simulink model "CM690A_HwAg0Meas"  (R2013b)
settings: Solver=FixedStepDiscrete  SolverMode=SingleTasking  StartTime=0.0  StopTime=22  FixedStep=0.002  RelTol=1e-3
undefined symbols (not defined in the file): ELECGLBPRM_DEGPERREV_DEGPERREV_F32, ELECGLBPRM_HWAGCENTROFFS_HWDEG_F32, ELECGLBPRM_HWAGSATNLOWRLIM_HWDEG_F32, ELECGLBPRM_HWAGSATNUPPRLIM_HWDEG_F32, ELECGLBPRM_HWAGSCA_ULS_F32, ELECGLBPRM_HWAGSPURGEARRAT_ULS_F32, ELECGLBPRM_HWAGSPURTORINGGEARRATSNSR0_ULS_F32, ELECGLBPRM_HWAGSPURTORINGGEARRATSNSR1_ULS_F32, ELECGLBPRM_NOFLT_CNT_U08, ELECGLBPRM_OFFSTRIMNOTPRFMD_CNT_U08, ELECGLBPRM_PRTCLFLT_CNT_U08, ELECGLBPRM_SKIPSTEPFLT_CNT_U08, ELECGLBPRM_SNSRINTFLT_CNT_U08, ELECGLBPRM_VRNRERRFLT_CNT_U08, FLTINJ_HWAG0MEAS_HWAG0, FLTINJ_HWAG0MEAS_TESTOK, HwAg0IfFlt, HwAg0MeasHwAg0IfFltFailStep, HwAg0MeasHwAg0IfFltPassStep, HwAg0MeasHwAg0Snsr0PrtclFltFailStep, HwAg0MeasHwAg0Snsr0PrtclFltPassStep, HwAg0MeasHwAg0Snsr1PrtclFltFailStep, HwAg0MeasHwAg0Snsr1PrtclFltPassStep, HwAg0MeasSnsr0Rev, HwAg0MeasSnsr1Rev, HwAg0MeasStep, HwAg0MeasVrnrErrThd, HwAg0MfgFlt, HwAg0Snsr0PrtclFlt, HwAg0Snsr1PrtclFlt, HWAG10THTOOTHTRIG_CNT_U08, HWAG11THTOOTHTRIG_CNT_U08, NtcSts1, sigbuilder_block, SigQlfr1
libraries: simulink x30, NxtrNvM x3
(part 2 of 5)

== system CM690A_HwAg0Meas/HwAg0Meas/HwAg0MeasPer2 ==
  note: Follow below steps in same order:
      |
      | 1. Check the Sensor Seq Number
      |    1a. Check Sensor Seq Number Logic first
      |    1b. Execute RawHwAgRead
      |    1c. Clear RSENT4CSC = 2046U;
      |    1d. FRS Flag Check: If the RegInpRSENT4FRS==1,  Read the RegInpRSENT4FND
      |
      | Design Note: Registers Read must be done once only. (Pl. see Design Rational Section for detail)
  RegInpRSENT4CS : Inport
  RegInpRSENT4FRXD : Inport  Port=2
  RegInpRSENT4FRS : Inport  Port=3
  RegInpRSENT4FND : Inport  Port=4
  function : TriggerPort  TriggerType=function-call
  Constant : Constant  Value=HWAG10THTOOTHTRIG_CNT_U08
      settings: AttributesFormatString=%<Value>.EngVal = 1
  CopyRight2 : Subsystem  Description=|  mask(Copyright Information){none=on}
      | Copyright info block.                                               
      |                                                                     
      | Place copyright information at the top of every subsystem in design.
      mask prompts: none "No parameters"
      mask help: Place copyright information at the top of every subsystem in design.
      mask Display:
      | NxtrConf = 'Nexteer Confidential';
      | 
      | sys = bdroot; %handle for the current model ("system")
      | first = get_param(sys,'Created');
      | first = first(end-3:end);  %year is last four digits
      | 
      | last = get_param(sys,'LastModifiedDate');
      | if isempty(last)
      |     last = datestr(now,'yyyy');
      | else
      |     last = last(end-3:end);
      | end
      | 
      | if strcmp(first,last)
      |     fprintf('%s -- Copyright %s Nexteer',NxtrConf,first)
      | else
      |     fprintf('%s -- %s%s- %s Nexteer',NxtrConf,char(169),first,last)
      | end
  Data Store Read1 : DataStoreRead  DataStoreName=HwAg0SnsrTrigNr
  If2 : If  RequirementInfo={} %GIDa_6155bf13_cddb_4606_817f_19ff0f92aa5f  NumInputs=2  IfExpression=u1 == u2
  Merge : Merge
  Merge1 : Merge
  Snsr0Read : Subsystem  RequirementInfo={} %GIDa_2ab6b8fe_3fe5_46cd_839a_e0a0bedc927a  TreatAsAtomicUnit=on
  Snsr0Read1 : Subsystem  RequirementInfo={} %GIDa_de6d45b7_1330_48a8_8a4c_631b6b0e9694  TreatAsAtomicUnit=on
  HwAg0Snsr0Raw : Outport
  HwAg0Snsr0TestOk : Outport  Port=2
  wires:
  If2/1 -> Snsr0Read/Action
  RegInpRSENT4CS/1 -> Snsr0Read/1(RegInpRSENT4CS)
  RegInpRSENT4FRXD/1 -> Snsr0Read/2(RegInpRSENT4FRXD)
  RegInpRSENT4FRS/1 -> Snsr0Read/3(RegInpRSENT4FRS)
  RegInpRSENT4FND/1 -> Snsr0Read/4(RegInpRSENT4FND)
  Merge/1 -> HwAg0Snsr0Raw/1
  Merge1/1 -> HwAg0Snsr0TestOk/1
  If2/2 -> Snsr0Read1/Action
  Snsr0Read/1(HwAg0Snsr0Raw) -> Merge/1
  Snsr0Read1/1(HwAg0Snsr0Raw) -> Merge/2
  Snsr0Read/2(HwAg0Snsr0TestOk) -> Merge1/1
  Snsr0Read1/2(HwAg0Snsr0TestOk) -> Merge1/2
  Data Store Read1/1 -> If2/1
  Constant/1 -> If2/2

== system CM690A_HwAg0Meas/HwAg0Meas/HwAg0MeasPer3 ==
  note: Follow below steps in same order:
      |
      | 1. Check the Sensor Seq Number
      |    1a. Check Sensor Seq Number Logic first
      |    1b. Execute RawHwAgRead
      |    1c. Clear RSENT4CSC = 2046U;
      |    1d. FRS Flag Check: If the RegInpRSENT4FRS==1,  Read the RegInpRSENT4FND
      |    1e. SYNCHRONIZATION PULSE Logic
      |
      | Design Note: Registers Read must be done once only. (Pl. see Design Rational Section for detail)
  RegInpRSENT4CS : Inport
  RegInpRSENT4FRXD : Inport  Port=2
  RegInpRSENT4NRS : Inport  Port=3
  RegInpRSENT4FRS : Inport  Port=4
  RegInpRSENT4FND : Inport  Port=5
  function : TriggerPort  TriggerType=function-call
  Constant : Constant  Value=HWAG11THTOOTHTRIG_CNT_U08
      settings: AttributesFormatString=%<Value>.EngVal = 2
  CopyRight2 : Subsystem  Description=|  mask(Copyright Information){none=on}
      | Copyright info block.                                               
      |                                                                     
      | Place copyright information at the top of every subsystem in design.
      mask prompts: none "No parameters"
      mask help: Place copyright information at the top of every subsystem in design.
      mask Display:
      | NxtrConf = 'Nexteer Confidential';
      | 
      | sys = bdroot; %handle for the current model ("system")
      | first = get_param(sys,'Created');
      | first = first(end-3:end);  %year is last four digits
      | 
      | last = get_param(sys,'LastModifiedDate');
      | if isempty(last)
      |     last = datestr(now,'yyyy');
      | else
      |     last = last(end-3:end);
      | end
      | 
      | if strcmp(first,last)
      |     fprintf('%s -- Copyright %s Nexteer',NxtrConf,first)
      | else
      |     fprintf('%s -- %s%s- %s Nexteer',NxtrConf,char(169),first,last)
      | end
  Data Store Read1 : DataStoreRead  DataStoreName=HwAg0SnsrTrigNr
  If1 : If  RequirementInfo={} %GIDa_c79673b4_d970_4e41_9a6f_d8dafcbbb0e1  NumInputs=2  IfExpression=u1 == u2
  Merge : Merge
  Merge1 : Merge
  Snsr1Read : Subsystem  RequirementInfo={} %GIDa_92d913f1_b7bc_4c95_8b6b_3f9b1805b54a  TreatAsAtomicUnit=on
  Snsr1Read1 : Subsystem  RequirementInfo={} %GIDa_e52a39b1_4a11_411e_af63_e5cd3b1f5705  TreatAsAtomicUnit=on
  HwAg0Snsr1Raw1 : Outport
  HwAg0Snsr1TestOk1 : Outport  Port=2
  wires:
  If1/2 -> Snsr1Read1/Action
  If1/1 -> Snsr1Read/Action
  RegInpRSENT4CS/1 -> Snsr1Read/1(RegInpRSENT4CS)
  RegInpRSENT4FRXD/1 -> Snsr1Read/2(RegInpRSENT4FRXD)
  RegInpRSENT4NRS/1 -> Snsr1Read/3(RegInpRSENT4NRS)
  RegInpRSENT4FRS/1 -> Snsr1Read/4(RegInpRSENT4FRS)
  RegInpRSENT4FND/1 -> Snsr1Read/5(RegInpRSENT4FND)
  Snsr1Read/1(HwAg0Snsr1Raw1) -> Merge/1
  Snsr1Read1/1(HwAg0Snsr1Raw) -> Merge/2
  Snsr1Read/2(HwAg0Snsr1TestOk1) -> Merge1/1
  Snsr1Read1/2(HwAg0Snsr1TestOk) -> Merge1/2
  Merge1/1 -> HwAg0Snsr1TestOk1/1
  Merge/1 -> HwAg0Snsr1Raw1/1
  Data Store Read1/1 -> If1/1
  Constant/1 -> If1/2

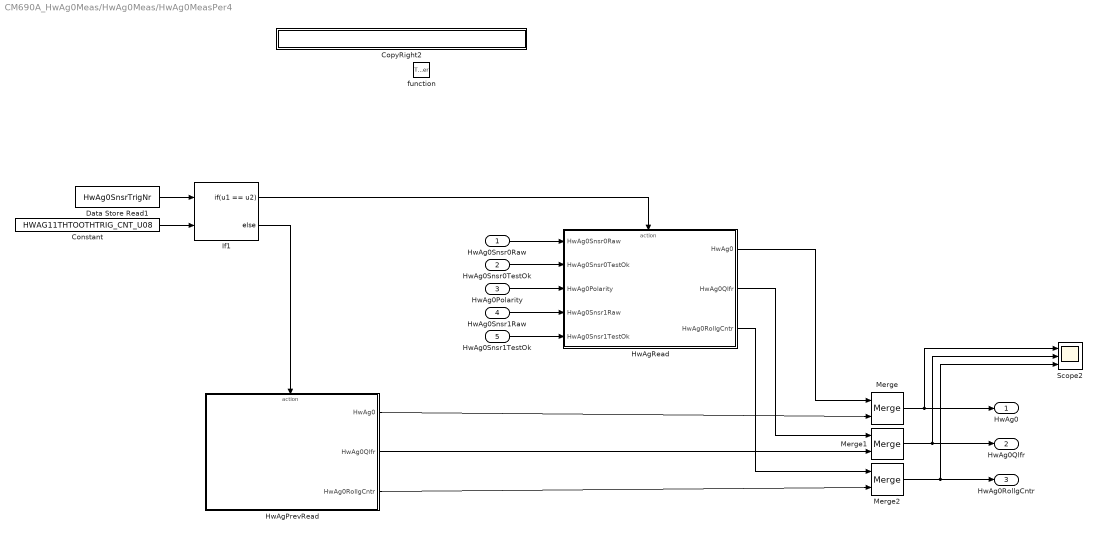
== system CM690A_HwAg0Meas/HwAg0Meas/HwAg0MeasPer4 ==
  HwAg0Snsr0Raw : Inport
  HwAg0Snsr0TestOk : Inport  Port=2
  HwAg0Polarity : Inport  Port=3
  HwAg0Snsr1Raw : Inport  Port=4
  HwAg0Snsr1TestOk : Inport  Port=5
  function : TriggerPort  TriggerType=function-call
  Constant : Constant  Value=HWAG11THTOOTHTRIG_CNT_U08
      settings: AttributesFormatString=%<Value>.EngVal = 2
  CopyRight2 : Subsystem  Description=|  mask(Copyright Information){none=on}
      | Copyright info block.                                               
      |                                                                     
      | Place copyright information at the top of every subsystem in design.
      mask prompts: none "No parameters"
      mask help: Place copyright information at the top of every subsystem in design.
      mask Display:
      | NxtrConf = 'Nexteer Confidential';
      | 
      | sys = bdroot; %handle for the current model ("system")
      | first = get_param(sys,'Created');
      | first = first(end-3:end);  %year is last four digits
      | 
      | last = get_param(sys,'LastModifiedDate');
      | if isempty(last)
      |     last = datestr(now,'yyyy');
      | else
      |     last = last(end-3:end);
      | end
      | 
      | if strcmp(first,last)
      |     fprintf('%s -- Copyright %s Nexteer',NxtrConf,first)
      | else
      |     fprintf('%s -- %s%s- %s Nexteer',NxtrConf,char(169),first,last)
      | end
  Data Store Read1 : DataStoreRead  DataStoreName=HwAg0SnsrTrigNr
  HwAgPrevRead : Subsystem  RequirementInfo={} %GIDa_7375e5dd_6ef3_4731_8150_c23cbc79327b  TreatAsAtomicUnit=on
  HwAgRead : Subsystem  RequirementInfo={} %GIDa_49b889d0_5e4f_426b_aa27_45e0ea96525b  TreatAsAtomicUnit=on
  If1 : If  RequirementInfo={} %GIDa_424aef36_26a1_41c7_8cb5_430e6f82d644  NumInputs=2  IfExpression=u1 == u2
  Merge : Merge
  Merge1 : Merge
  Merge2 : Merge
  Scope2 : Scope  NumInputPorts=3
      settings: TimeRange=22  YMin=-900~0~1  YMax=900~275~2  SaveName=ScopeData6
  HwAg0 : Outport  RequirementInfo={} %GIDa_a55d0ad3_e601_49c7_b914_9c4e7bab7fda
  HwAg0Qlfr : Outport  RequirementInfo={'linktype_rmi_doors' '0000cf45 (/ESG Group/FDD Module Requirements/EA4 Specific/CM690A_HwAg0Meas)' '#CM690A_30' 'true' 'REQ: CM690A_30' '' } %GIDa_08dc6d09_800d_4647_82e3_4af412467949  Port=2
  HwAg0RollgCntr : Outport  RequirementInfo={'linktype_rmi_doors' '0000cf45 (/ESG Group/FDD Module Requirements/EA4 Specific/CM690A_HwAg0Meas)' '#CM690A_31' 'true' 'REQ: CM690A_31' '' } %GIDa_3c51bdf7_5d2b_4414_9b3f_5b588ccc6872  Port=3
  wires:
  If1/2 -> HwAgPrevRead/Action
  If1/1 -> HwAgRead/Action
  HwAgRead/1(HwAg0) -> Merge/1
  HwAgPrevRead/1(HwAg0) -> Merge/2
  HwAgRead/2(HwAg0Qlfr) -> Merge1/1
  HwAgPrevRead/2(HwAg0Qlfr) -> Merge1/2
  HwAgPrevRead/3(HwAg0RollgCntr) -> Merge2/2
  HwAgRead/3(HwAg0RollgCntr) -> Merge2/1
  Merge/1 -> Scope2/1, HwAg0/1
  Merge1/1 -> Scope2/2, HwAg0Qlfr/1
  Merge2/1 -> Scope2/3, HwAg0RollgCntr/1
  HwAg0Snsr1Raw/1 -> HwAgRead/4(HwAg0Snsr1Raw)
  HwAg0Polarity/1 -> HwAgRead/3(HwAg0Polarity)
  HwAg0Snsr1TestOk/1 -> HwAgRead/5(HwAg0Snsr1TestOk)
  HwAg0Snsr0TestOk/1 -> HwAgRead/2(HwAg0Snsr0TestOk)
  HwAg0Snsr0Raw/1 -> HwAgRead/1(HwAg0Snsr0Raw)
  Data Store Read1/1 -> If1/1
  Constant/1 -> If1/2

== system CM690A_HwAg0Meas/HwAg0Meas/HwAg0MeasPer5 ==
  note: Information Only:
      | - Trim not performed Ntc
  function : TriggerPort  TriggerType=function-call
  Constant : Constant  Value=HwAg0MfgFlt
  CopyRight2 : Subsystem  Description=|  mask(Copyright Information){none=on}
      | Copyright info block.                                               
      |                                                                     
      | Place copyright information at the top of every subsystem in design.
      mask prompts: none "No parameters"
      mask help: Place copyright information at the top of every subsystem in design.
      mask Display:
      | NxtrConf = 'Nexteer Confidential';
      | 
      | sys = bdroot; %handle for the current model ("system")
      | first = get_param(sys,'Created');
      | first = first(end-3:end);  %year is last four digits
      | 
      | last = get_param(sys,'LastModifiedDate');
      | if isempty(last)
      |     last = datestr(now,'yyyy');
      | else
      |     last = last(end-3:end);
      | end
      | 
      | if strcmp(first,last)
      |     fprintf('%s -- Copyright %s Nexteer',NxtrConf,first)
      | else
      |     fprintf('%s -- %s%s- %s Nexteer',NxtrConf,char(169),first,last)
      | end
  Data Store Read1 : DataStoreRead  DataStoreName=HwAg0OffsTrimPrfmdSts
  Ground : Ground
  If : If  IfExpression=(u1 ~= 0)
  If Action Subsystem : Subsystem  RequirementInfo={'linktype_rmi_doors' '0000cf45 (/ESG Group/FDD Module Requirements/EA4 Specific/CM690A_HwAg0Meas)' '#CM690A_107' 'true' 'REQ: CM690A_107' '' } %GIDa_93c0c2f6_38ee_4160_b051_f0ab663f9dc9  TreatAsAtomicUnit=on
  If Action Subsystem1 : Subsystem  RequirementInfo={'linktype_rmi_doors' '0000cf45 (/ESG Group/FDD Module Requirements/EA4 Specific/CM690A_HwAg0Meas)' '#CM690A_104' 'true' 'REQ: CM690A_104' '' } %GIDa_fa6d762f_0a06_4ac8_8aec_4f8d74e26f90  TreatAsAtomicUnit=on
  Merge : Merge
  Merge1 : Merge
  Scope : Scope  NumInputPorts=2
      settings: YMin=-5~-5  YMax=5~5  SaveName=ScopeData3
  SetNtcSts : Subsystem  RequirementInfo={'linktype_rmi_doors' '0000cf45 (/ESG Group/FDD Module Requirements/EA4 Specific/CM690A_HwAg0Meas)' '#CM690A_100' 'true' 'REQ: CM690A_100' '' } %GIDa_9e3edb63_7888_44cf_a718_771f9129b5ad
  wires:
  Ground/1 -> SetNtcSts/4(DebStep)
  Constant/1 -> SetNtcSts/1(NtcNr)
  Data Store Read1/1 -> If/1
  If/1 -> If Action Subsystem/Action
  If/2 -> If Action Subsystem1/Action
  If Action Subsystem/1(ParamByte) -> Merge/1
  If Action Subsystem1/1(ParamByte) -> Merge/2
  If Action Subsystem/2(TestOk) -> Merge1/1
  If Action Subsystem1/2(TestOk) -> Merge1/2
  Merge/1 -> Scope/1, SetNtcSts/2(NtcStInfo)  "ParamByte"
  Merge1/1 -> Scope/2, SetNtcSts/3(NtcSts)  "TestOk"

== system CM690A_HwAg0Meas/Simulated_Input/CopyRight2 ==

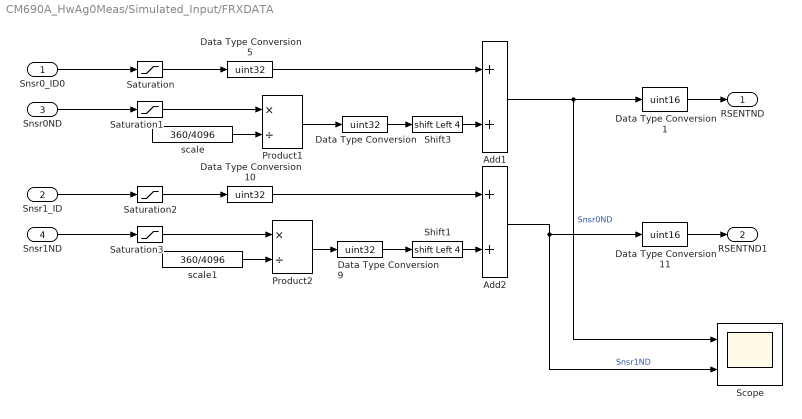
== system CM690A_HwAg0Meas/Simulated_Input/FRXDATA ==
  Snsr0_ID0 : Inport
  Snsr1_ID : Inport  Port=2
  Snsr0ND : Inport  Port=3
  Snsr1ND : Inport  Port=4
  Add1 : Sum
  Add2 : Sum
  Data Type Conversion : DataTypeConversion  OutDataTypeStr=uint32
  Data Type Conversion1 : DataTypeConversion  OutDataTypeStr=uint16
  Data Type Conversion10 : DataTypeConversion  OutDataTypeStr=uint32  SaturateOnIntegerOverflow=on
  Data Type Conversion11 : DataTypeConversion  OutDataTypeStr=uint16
  Data Type Conversion5 : DataTypeConversion  OutDataTypeStr=uint32
  Data Type Conversion9 : DataTypeConversion  OutDataTypeStr=uint32
  Product1 : Product  Inputs=*/
  Product2 : Product  Inputs=*/
  Saturation : Saturate  UpperLimit=1  LowerLimit=0
  Saturation1 : Saturate  UpperLimit=360  LowerLimit=0
  Saturation2 : Saturate  UpperLimit=1  LowerLimit=0
  Saturation3 : Saturate  UpperLimit=360  LowerLimit=0
  Scope : Scope  NumInputPorts=2
      settings: YMin=1.02005e+09~0  YMax=1.12743e+09~6e+08
  Shift1 : ArithShift  BitShiftNumber=4  BitShiftDirection=Left
  Shift3 : ArithShift  BitShiftNumber=4  BitShiftDirection=Left
  scale : Constant  Value=360/4096
  scale1 : Constant  Value=360/4096
  RSENTND : Outport
  RSENTND1 : Outport  Port=2
  wires:
  Snsr0ND/1 -> Saturation1/1
  scale/1 -> Product1/2
  Product1/1 -> Data Type Conversion/1
  Data Type Conversion1/1 -> RSENTND/1
  Snsr0_ID0/1 -> Saturation/1
  Data Type Conversion5/1 -> Add1/1
  Data Type Conversion/1 -> Shift3/1
  Add1/1 -> Scope/1, Data Type Conversion1/1  "Snsr0ND"
  Snsr1ND/1 -> Saturation3/1
  scale1/1 -> Product2/2
  Product2/1 -> Data Type Conversion9/1
  Snsr1_ID/1 -> Saturation2/1
  Data Type Conversion10/1 -> Add2/1
  Data Type Conversion9/1 -> Shift1/1
  Data Type Conversion11/1 -> RSENTND1/1
  Add2/1 -> Data Type Conversion11/1, Scope/2  "Snsr1ND"
  Saturation/1 -> Data Type Conversion5/1
  Saturation1/1 -> Product1/1
  Saturation2/1 -> Data Type Conversion10/1
  Saturation3/1 -> Product2/1
  Shift3/1 -> Add1/2
  Shift1/1 -> Add2/2

== system CM690A_HwAg0Meas/Simulated_Input/FRXDATA1 ==
  Snsr0_CS : Inport
  Snsr1_CS : Inport  Port=2
  Snsr0_FRS : Inport  Port=3
  Snsr1_FRS : Inport  Port=4
  Add1 : Sum
  Add2 : Sum
  Data Type Conversion{,1,5,9,11} (5 alike) : DataTypeConversion  OutDataTypeStr=uint32
  Data Type Conversion10 : DataTypeConversion  OutDataTypeStr=uint32  SaturateOnIntegerOverflow=on
  Scope : Scope  NumInputPorts=2
      settings: YMin=1.02005e+09~0  YMax=1.12743e+09~6e+08
  Shift1 : ArithShift  BitShiftNumber=1  BitShiftDirection=Left
  Shift3 : ArithShift  BitShiftNumber=1  BitShiftDirection=Left
  Snsr0CS : Outport
  Snsr1CS : Outport  Port=2
  wires:
  Data Type Conversion9/1 -> Add2/2
  Data Type Conversion/1 -> Add1/2
  Snsr1_CS/1 -> Data Type Conversion10/1
  Snsr0_CS/1 -> Data Type Conversion5/1
  Add2/1 -> Scope/2, Data Type Conversion11/1  "Snsr1ND"
  Data Type Conversion11/1 -> Snsr1CS/1
  Data Type Conversion10/1 -> Shift1/1
  Add1/1 -> Data Type Conversion1/1, Scope/1  "Snsr0ND"
  Data Type Conversion5/1 -> Shift3/1
  Data Type Conversion1/1 -> Snsr0CS/1
  Snsr0_FRS/1 -> Data Type Conversion/1
  Snsr1_FRS/1 -> Data Type Conversion9/1
  Shift3/1 -> Add1/1
  Shift1/1 -> Add2/1

== system CM690A_HwAg0Meas/Simulated_Input/FRXDATA2 ==
  Snsr0_FCCN : Inport
  Snsr1_FCCN : Inport  Port=2
  Snsr0_Data : Inport  Port=3
  Snsr1_Data : Inport  Port=4
  Add1 : Sum
  Add2 : Sum
  Data Type Conversion{,1,5,9,11} (5 alike) : DataTypeConversion  OutDataTypeStr=uint32
  Data Type Conversion10 : DataTypeConversion  OutDataTypeStr=uint32  SaturateOnIntegerOverflow=on
  Scope : Scope  NumInputPorts=2
      settings: YMin=1.02005e+09~0  YMax=1.12743e+09~6e+08
  Shift1 : ArithShift  BitShiftNumber=28  BitShiftDirection=Left
  Shift3 : ArithShift  BitShiftNumber=28  BitShiftDirection=Left
  Snsr0FRXD : Outport
  Snsr1FRXD : Outport  Port=2
  wires:
  Shift1/1 -> Add2/1
  Shift3/1 -> Add1/1
  Snsr1_Data/1 -> Data Type Conversion9/1
  Snsr0_Data/1 -> Data Type Conversion/1
  Data Type Conversion1/1 -> Snsr0FRXD/1
  Data Type Conversion5/1 -> Shift3/1
  Add1/1 -> Scope/1, Data Type Conversion1/1  "Snsr0ND"
  Data Type Conversion10/1 -> Shift1/1
  Data Type Conversion11/1 -> Snsr1FRXD/1
  Add2/1 -> Data Type Conversion11/1, Scope/2  "Snsr1ND"
  Snsr0_FCCN/1 -> Data Type Conversion5/1
  Snsr1_FCCN/1 -> Data Type Conversion10/1
  Data Type Conversion/1 -> Add1/2
  Data Type Conversion9/1 -> Add2/2

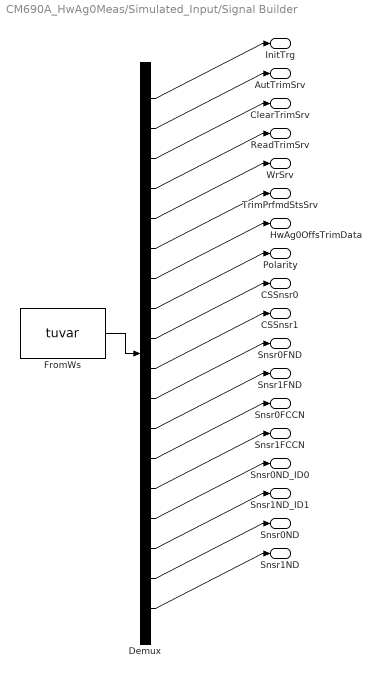
== system CM690A_HwAg0Meas/Simulated_Input/Signal Builder ==
  Demux : Demux  Tag=STV Demux  Outputs=18
  FromWs : FromWorkspace  Tag=STV FromWs  VariableName=tuvar  SampleTime=0  OutputAfterFinalValue=Holding final value
      SigBuilderData=|
      | common.afterFinalStr = 'Hold final value'
      | common.sampleTime = '0'
      | dataSet(1).timeRange = [0 22]
      | dataSet(1).name = 'IdealSignal'
      | dataSet(2).timeRange = [0 22]
      | dataSet(2).name = 'Faults'
      | dataSet(3).timeRange = [0 22]
      | dataSet(3).name = 'Service'
      | dataSet(4).timeRange = [0 22]
      | dataSet(4).name = 'RollOver'
      | sbobj.Groups(1).Name = 'IdealSignal'
      | sbobj.Groups(1).Signals(1).Name = 'InitTrg'
      | sbobj.Groups(1).Signals(1).XData = [0 0.02 0.02 0.06 0.06 22]
      | sbobj.Groups(1).Signals(1).YData = [0 0 1 1 0 0]
      | sbobj.Groups(1).Signals(2).Name = 'AutTrimSrv'
      | sbobj.Groups(1).Signals(2).XData = [0 22]
      | sbobj.Groups(1).Signals(2).YData = [0 0]
      | sbobj.Groups(1).Signals(3).Name = 'ClearTrimSrv'
      | sbobj.Groups(1).Signals(3).XData = [0 22]
      | sbobj.Groups(1).Signals(3).YData = [0 0]
      | sbobj.Groups(1).Signals(4).Name = 'ReadTrimSrv'
      | sbobj.Groups(1).Signals(4).XData = [0 22]
      | sbobj.Groups(1).Signals(4).YData = [0 0]
      | sbobj.Groups(1).Signals(5).Name = 'WrSrv'
      | sbobj.Groups(1).Signals(5).XData = [0 0.04 0.04 0.08 0.08 22]
      | sbobj.Groups(1).Signals(5).YData = [0 0 1 1 0 0]
      | sbobj.Groups(1).Signals(6).Name = 'TrimPrfmdStsSrv'
      | sbobj.Groups(1).Signals(6).XData = [0 22]
      | sbobj.Groups(1).Signals(6).YData = [0 0]
      | sbobj.Groups(1).Signals(7).Name = 'HwAg0OffsTrimData'
      | sbobj.Groups(1).Signals(7).XData = [0 22]
      | sbobj.Groups(1).Signals(7).YData = [0 0]
      | sbobj.Groups(1).Signals(8).Name = 'Polarity'
      | sbobj.Groups(1).Signals(8).XData = [0 22]
      | sbobj.Groups(1).Signals(8).YData = [1 1]
      | sbobj.Groups(1).Signals(9).Name = 'CSSnsr0'
      | sbobj.Groups(1).Signals(9).XData = [0 22]
      | sbobj.Groups(1).Signals(9).YData = [0 0]
      | sbobj.Groups(1).Signals(10).Name = 'CSSnsr1'
      | sbobj.Groups(1).Signals(10).XData = [0 22]
      | sbobj.Groups(1).Signals(10).YData = [0 0]
      | sbobj.Groups(1).Signals(11).Name = 'Snsr0FND'
      | sbobj.Groups(1).Signals(11).XData = [0 22]
      | sbobj.Groups(1).Signals(11).YData = [1 1]
      | sbobj.Groups(1).Signals(12).Name = 'Snsr1FND'
      | sbobj.Groups(1).Signals(12).XData = [0 22]
      | sbobj.Groups(1).Signals(12).YData = [1 1]
      | sbobj.Groups(1).Signals(13).Name = 'Snsr0FCCN'
      | sbobj.Groups(1).Signals(13).XData = [0 22]
      | sbobj.Groups(1).Signals(13).YData = [0 0]
      | sbobj.Groups(1).Signals(14).Name = 'Snsr1FCCN'
      | sbobj.Groups(1).Signals(14).XData = [0 22]
      | sbobj.Groups(1).Signals(14).YData = [0 0]
      | sbobj.Groups(1).Signals(15).Name = 'Snsr0ND_ID0'
      | sbobj.Groups(1).Signals(15).XData = [0 22]
      | sbobj.Groups(1).Signals(15).YData = [0 0]
      | sbobj.Groups(1).Signals(16).Name = 'Snsr1ND_ID1'
      | sbobj.Groups(1).Signals(16).XData = [0 22]
      | sbobj.Groups(1).Signals(16).YData = [1 1]
      | sbobj.Groups(1).Signals(17).Name = 'Snsr0ND'
      | sbobj.Groups(1).Signals(17).XData = [0 2 2 4 4 6 6 8 8 10 10 12 12 14 14 16 16 18 18 20 20 22]
      | sbobj.Groups(1).Signals(17).YData = [0 359.9 0 359.9 0 359.9 0 359.9 0 359.9 0 359.9 0 359.9 0 359.9 0 359.9 0 359.9 0 359.9]
      | sbobj.Groups(1).Signals(18).Name = 'Snsr1ND'
      | sbobj.Groups(1).Signals(18).XData = [0 2.2000022 2.2000022 4.4000044 4.4000044 6.60000660001 6.60000660001 8.80000880001 8.80000880001 11.000011 11.000011 13.2000132 13.2000132 15.4000154 15.4000154 17.6000176 17.6000176 19.8000198 19.8000198 22]
      | sbobj.Groups(1).Signals(18).YData = [0 359.9 0 359.9 0 359.9 0 359.9 0 359.9 0 359.9 0 359.9 0 359.9 0 359.9 0 359.896401]
      | sbobj.Groups(1).TimeRange = [0 22]
      | sbobj.Groups(2).Name = 'Faults'
      | sbobj.Groups(2).Signals(1).Name = 'InitTrg'
      | sbobj.Groups(2).Signals(1).XData = [0 0.02 0.02 0.06 0.06 22]
      | sbobj.Groups(2).Signals(1).YData = [0 0 1 1 0 0]
      | sbobj.Groups(2).Signals(2).Name = 'AutTrimSrv'
      | sbobj.Groups(2).Signals(2).XData = [0 22]
      | sbobj.Groups(2).Signals(2).YData = [0 0]
      | sbobj.Groups(2).Signals(3).Name = 'ClearTrimSrv'
      | sbobj.Groups(2).Signals(3).XData = [0 22]
      | sbobj.Groups(2).Signals(3).YData = [0 0]
      | sbobj.Groups(2).Signals(4).Name = 'ReadTrimSrv'
      | sbobj.Groups(2).Signals(4).XData = [0 22]
      | sbobj.Groups(2).Signals(4).YData = [0 0]
      | sbobj.Groups(2).Signals(5).Name = 'WrSrv'
      | sbobj.Groups(2).Signals(5).XData = [0 0.06 0.06 0.12 0.12 22]
      | sbobj.Groups(2).Signals(5).YData = [0 0 1 1 0 0]
      | sbobj.Groups(2).Signals(6).Name = 'TrimPrfmdStsSrv'
      | sbobj.Groups(2).Signals(6).XData = [0 22]
      | sbobj.Groups(2).Signals(6).YData = [0 0]
      | sbobj.Groups(2).Signals(7).Name = 'HwAg0OffsTrimData'
      | sbobj.Groups(2).Signals(7).XData = [0 22]
      | sbobj.Groups(2).Signals(7).YData = [0 0]
      | sbobj.Groups(2).Signals(8).Name = 'Polarity'
      | sbobj.Groups(2).Signals(8).XData = [0 11 11 22]
      | sbobj.Groups(2).Signals(8).YData = [-1 -1 1 1]
      | sbobj.Groups(2).Signals(9).Name = 'CSSnsr0'
      | sbobj.Groups(2).Signals(9).XData = [0 2.54 2.54 2.88 2.88 22]
      | sbobj.Groups(2).Signals(9).YData = [0 0 2 2 0 0]
      | sbobj.Groups(2).Signals(10).Name = 'CSSnsr1'
      | sbobj.Groups(2).Signals(10).XData = [0 4.36 4.36 4.78 4.78 22]
      | sbobj.Groups(2).Signals(10).YData = [0 0 2 2 0 0]
      | sbobj.Groups(2).Signals(11).Name = 'Snsr0FND'
      | sbobj.Groups(2).Signals(11).XData = [0 14.54 14.54 14.78 14.78 22]
      | sbobj.Groups(2).Signals(11).YData = [1 1 0 0 1 1]
      | sbobj.Groups(2).Signals(12).Name = 'Snsr1FND'
      | sbobj.Groups(2).Signals(12).XData = [0 15.66 15.66 15.94 15.94 22]
      | sbobj.Groups(2).Signals(12).YData = [1 1 0 0 1 1]
      | sbobj.Groups(2).Signals(13).Name = 'Snsr0FCCN'
      | sbobj.Groups(2).Signals(13).XData = [0 12.02 12.02 12.26 12.26 22]
      | sbobj.Groups(2).Signals(13).YData = [0 0 1 1 0 0]
      | sbobj.Groups(2).Signals(14).Name = 'Snsr1FCCN'
      | sbobj.Groups(2).Signals(14).XData = [0 12.92 12.92 13.2 13.2 22]
      | sbobj.Groups(2).Signals(14).YData = [0 0 2 2 0 0]
      | sbobj.Groups(2).Signals(15).Name = 'Snsr0ND_ID0'
      | sbobj.Groups(2).Signals(15).XData = [0 6.46 6.46 6.8 6.8 22]
      | sbobj.Groups(2).Signals(15).YData = [0 0 1 1 0 0]
      | sbobj.Groups(2).Signals(16).Name = 'Snsr1ND_ID1'
      | sbobj.Groups(2).Signals(16).XData = [0 8.8 8.8 9.32 9.32 22]
      | sbobj.Groups(2).Signals(16).YData = [1 1 0 0 1 1]
      | sbobj.Groups(2).Signals(17).Name = 'Snsr0ND'
      | sbobj.Groups(2).Signals(17).XData = [0 2 2 4 4 6 6 8 8 10 10 12 12 14 14 16 16 18 18 20 20 22]
      | sbobj.Groups(2).Signals(17).YData = [0 359.9 0 359.9 0 359.9 0 359.9 0 359.9 0 359.9 0 359.9 0 359.9 0 359.9 0 359.9 0 350]
      | sbobj.Groups(2).Signals(18).Name = 'Snsr1ND'
      | sbobj.Groups(2).Signals(18).XData = [0 2.2000022 2.2000022 4.4000044 4.4000044 6.60000660001 6.60000660001 8.80000880001 8.80000880001 11.000011 11.000011 13.2000132 13.2000132 15.4000154 15.4000154 17.6000176 17.6000176 20 20 22]
      | sbobj.Groups(2).Signals(18).YData = [0 359.9 0 359.9 0 359.9 0 359.9 0 359.9 0 359.9 0 359.9 0 359.9 0 359.9 0 350]
      | sbobj.Groups(2).TimeRange = [0 22]
      | sbobj.Groups(3).Name = 'Service'
      | sbobj.Groups(3).Signals(1).Name = 'InitTrg'
      | sbobj.Groups(3).Signals(1).XData = [0 0.02 0.02 0.06 0.06 22]
      | sbobj.Groups(3).Signals(1).YData = [0 0 1 1 0 0]
      | sbobj.Groups(3).Signals(2).Name = 'AutTrimSrv'
      | sbobj.Groups(3).Signals(2).XData = [0 0.58 0.58 0.68 0.68 16 16 16.1 16.1 22]
      | sbobj.Groups(3).Signals(2).YData = [0 0 1 1 0 0 1 1 0 0]
      | sbobj.Groups(3).Signals(3).Name = 'ClearTrimSrv'
      | sbobj.Groups(3).Signals(3).XData = [0 0.34 4.1 4.1 4.16 4.16 9.98 9.98 10.06 10.06 22]
      | sbobj.Groups(3).Signals(3).YData = [0 0 0 1 1 0 0 1 1 0 0]
      | sbobj.Groups(3).Signals(4).Name = 'ReadTrimSrv'
      | sbobj.Groups(3).Signals(4).XData = [0 1.24 1.24 1.32 1.32 4.62 4.62 4.7 4.7 6.84 6.84 6.92 6.92 10.38 10.38 10.46 10.46 16.72 16.72 16.8 16.8 22]
      | sbobj.Groups(3).Signals(4).YData = [0 0 1 1 0 0 1 1 0 0 1 1 0 0 1 1 0 0 1 1 0 0]
      | sbobj.Groups(3).Signals(5).Name = 'WrSrv'
      | sbobj.Groups(3).Signals(5).XData = [0 6.22 6.22 6.3 6.3 22]
      | sbobj.Groups(3).Signals(5).YData = [0 0 1 1 0 0]
      | sbobj.Groups(3).Signals(6).Name = 'TrimPrfmdStsSrv'
      | sbobj.Groups(3).Signals(6).XData = [0 1.24 1.24 1.32 1.32 4.64 4.64 4.7 4.7 6.84 6.84 6.92 6.92 10.64 10.64 10.72 10.72 16.74 16.74 16.82 16.82 22]
      | sbobj.Groups(3).Signals(6).YData = [0 0 1 1 0 0 1 1 0 0 1 1 0 0 1 1 0 0 1 1 0 0]
      | sbobj.Groups(3).Signals(7).Name = 'HwAg0OffsTrimData'
      | sbobj.Groups(3).Signals(7).XData = [0 0.4 5.4 5.4 11.16 11.16 22]
      | sbobj.Groups(3).Signals(7).YData = [0 0 0 300 300 0 0]
      | sbobj.Groups(3).Signals(8).Name = 'Polarity'
      | sbobj.Groups(3).Signals(8).XData = [0 22]
      | sbobj.Groups(3).Signals(8).YData = [1 1]
      | sbobj.Groups(3).Signals(9).Name = 'CSSnsr0'
      | sbobj.Groups(3).Signals(9).XData = [0 22]
      | sbobj.Groups(3).Signals(9).YData = [0 0]
      | sbobj.Groups(3).Signals(10).Name = 'CSSnsr1'
      | sbobj.Groups(3).Signals(10).XData = [0 22]
      | sbobj.Groups(3).Signals(10).YData = [0 0]
      | sbobj.Groups(3).Signals(11).Name = 'Snsr0FND'
      | sbobj.Groups(3).Signals(11).XData = [0 22]
      | sbobj.Groups(3).Signals(11).YData = [1 1]
      | sbobj.Groups(3).Signals(12).Name = 'Snsr1FND'
      | sbobj.Groups(3).Signals(12).XData = [0 22]
      | sbobj.Groups(3).Signals(12).YData = [1 1]
      | sbobj.Groups(3).Signals(13).Name = 'Snsr0FCCN'
      | sbobj.Groups(3).Signals(13).XData = [0 22]
      | sbobj.Groups(3).Signals(13).YData = [0 0]
      | sbobj.Groups(3).Signals(14).Name = 'Snsr1FCCN'
      | sbobj.Groups(3).Signals(14).XData = [0 22]
      | sbobj.Groups(3).Signals(14).YData = [0 0]
      | sbobj.Groups(3).Signals(15).Name = 'Snsr0ND_ID0'
      | sbobj.Groups(3).Signals(15).XData = [0 22]
      | sbobj.Groups(3).Signals(15).YData = [0 0]
      | sbobj.Groups(3).Signals(16).Name = 'Snsr1ND_ID1'
      | sbobj.Groups(3).Signals(16).XData = [0 22]
      | sbobj.Groups(3).Signals(16).YData = [1 1]
      | sbobj.Groups(3).Signals(17).Name = 'Snsr0ND'
      | sbobj.Groups(3).Signals(17).XData = [0 2 2 4 4 6 6 8 8 10 10 12 12 14 14 16 16 18 18 20 20 22]
      | sbobj.Groups(3).Signals(17).YData = [0 359.9 0 359.9 0 359.9 0 359.9 0 359.9 0 359.9 0 359.9 0 359.9 0 359.9 0 359.9 0 359.9]
      | sbobj.Groups(3).Signals(18).Name = 'Snsr1ND'
      | sbobj.Groups(3).Signals(18).XData = [0 2.2000022 2.2000022 4.4000044 4.4000044 6.60000660001 6.60000660001 8.80000880001 8.80000880001 11.000011 11.000011 13.2000132 13.2000132 15.4000154 15.4000154 17.6000176 17.6000176 19.8000198 19.8000198 22]
      | sbobj.Groups(3).Signals(18).YData = [0 359.9 0 359.9 0 359.9 0 359.9 0 359.9 0 359.9 0 359.9 0 359.9 0 359.9 0 359.896401]
      | sbobj.Groups(3).TimeRange = [0 22]
      | sbobj.Groups(4).Name = 'RollOver'
      | sbobj.Groups(4).Signals(1).Name = 'InitTrg'
      | sbobj.Groups(4).Signals(1).XData = [0 0.02 0.02 0.06 0.06 22]
      | sbobj.Groups(4).Signals(1).YData = [0 0 1 1 0 0]
      | sbobj.Groups(4).Signals(2).Name = 'AutTrimSrv'
      | sbobj.Groups(4).Signals(2).XData = [0 0.58 0.58 0.68 0.68 15.76 16.1 22]
      | sbobj.Groups(4).Signals(2).YData = [0 0 1 1 0 0 0 0]
      | sbobj.Groups(4).Signals(3).Name = 'ClearTrimSrv'
      | sbobj.Groups(4).Signals(3).XData = [0 22]
      | sbobj.Groups(4).Signals(3).YData = [0 0]
      | sbobj.Groups(4).Signals(4).Name = 'ReadTrimSrv'
      | sbobj.Groups(4).Signals(4).XData = [0 1.24 1.24 1.32 1.32 4.62 4.62 4.7 4.7 6.84 6.84 6.92 6.92 10.38 10.38 10.46 10.46 16.72 16.72 16.8 16.8 22]
      | sbobj.Groups(4).Signals(4).YData = [0 0 1 1 0 0 1 1 0 0 1 1 0 0 1 1 0 0 1 1 0 0]
      | sbobj.Groups(4).Signals(5).Name = 'WrSrv'
      | sbobj.Groups(4).Signals(5).XData = [0 22]
      | sbobj.Groups(4).Signals(5).YData = [0 0]
      | sbobj.Groups(4).Signals(6).Name = 'TrimPrfmdStsSrv'
      | sbobj.Groups(4).Signals(6).XData = [0 1.24 1.24 1.32 1.32 4.64 4.64 4.7 4.7 6.84 6.84 6.92 6.92 10.64 10.64 10.72 10.72 16.74 16.74 16.82 16.82 22]
      | sbobj.Groups(4).Signals(6).YData = [0 0 1 1 0 0 1 1 0 0 1 1 0 0 1 1 0 0 1 1 0 0]
      | sbobj.Groups(4).Signals(7).Name = 'HwAg0OffsTrimData'
      | sbobj.Groups(4).Signals(7).XData = [0 0.4 5.4 5.4 11.16 11.16 22]
      | sbobj.Groups(4).Signals(7).YData = [0 0 0 300 300 0 0]
      | sbobj.Groups(4).Signals(8).Name = 'Polarity'
      | sbobj.Groups(4).Signals(8).XData = [0 22]
      | sbobj.Groups(4).Signals(8).YData = [1 1]
      | sbobj.Groups(4).Signals(9).Name = 'CSSnsr0'
      | sbobj.Groups(4).Signals(9).XData = [0 22]
      | sbobj.Groups(4).Signals(9).YData = [0 0]
      | sbobj.Groups(4).Signals(10).Name = 'CSSnsr1'
      | sbobj.Groups(4).Signals(10).XData = [0 22]
      | sbobj.Groups(4).Signals(10).YData = [0 0]
      | sbobj.Groups(4).Signals(11).Name = 'Snsr0FND'
      | sbobj.Groups(4).Signals(11).XData = [0 22]
      | sbobj.Groups(4).Signals(11).YData = [1 1]
      | sbobj.Groups(4).Signals(12).Name = 'Snsr1FND'
      | sbobj.Groups(4).Signals(12).XData = [0 22]
      | sbobj.Groups(4).Signals(12).YData = [1 1]
      | sbobj.Groups(4).Signals(13).Name = 'Snsr0FCCN'
      | sbobj.Groups(4).Signals(13).XData = [0 22]
      | sbobj.Groups(4).Signals(13).YData = [0 0]
      | sbobj.Groups(4).Signals(14).Name = 'Snsr1FCCN'
      | sbobj.Groups(4).Signals(14).XData = [0 22]
      | sbobj.Groups(4).Signals(14).YData = [0 0]
      | sbobj.Groups(4).Signals(15).Name = 'Snsr0ND_ID0'
      | sbobj.Groups(4).Signals(15).XData = [0 22]
      | sbobj.Groups(4).Signals(15).YData = [0 0]
      | sbobj.Groups(4).Signals(16).Name = 'Snsr1ND_ID1'
      | sbobj.Groups(4).Signals(16).XData = [0 22]
      | sbobj.Groups(4).Signals(16).YData = [1 1]
      | sbobj.Groups(4).Signals(17).Name = 'Snsr0ND'
      | sbobj.Groups(4).Signals(17).XData = [0 2 2 4 4 6 6 8 8 10 10 12 12 14 14 16 16 18 18 20 20 22]
      | sbobj.Groups(4).Signals(17).YData = [0 359.9 0 359.9 0 359.9 0 359.9 0 359.9 0 359.9 0 359.9 0 359.9 0 359.9 0 359.9 0 359.9]
      | sbobj.Groups(4).Signals(18).Name = 'Snsr1ND'
      | sbobj.Groups(4).Signals(18).XData = [0 2.2000022 2.2000022 4.4000044 4.4000044 6.60000660001 6.60000660001 8.80000880001 8.80000880001 11.000011 11.000011 13.2000132 13.2000132 15.4000154 15.4000154 17.6000176 17.6000176 19.8000198 19.8000198 22]
      | sbobj.Groups(4).Signals(18).YData = [0 359.9 0 359.9 0 359.9 0 359.9 0 359.9 0 359.9 0 359.9 0 359.9 0 359.9 0 359.896401]
      | sbobj.Groups(4).TimeRange = [0 22]
  InitTrg : Outport  Tag=STV Outport
  AutTrimSrv : Outport  Tag=STV Outport  Port=2
  ClearTrimSrv : Outport  Tag=STV Outport  Port=3
  ReadTrimSrv : Outport  Tag=STV Outport  Port=4
  WrSrv : Outport  Tag=STV Outport  Port=5
  TrimPrfmdStsSrv : Outport  Tag=STV Outport  Port=6
  HwAg0OffsTrimData : Outport  Tag=STV Outport  Port=7
  Polarity : Outport  Tag=STV Outport  Port=8
  CSSnsr0 : Outport  Tag=STV Outport  Port=9
  CSSnsr1 : Outport  Tag=STV Outport  Port=10
  Snsr0FND : Outport  Tag=STV Outport  Port=11
  Snsr1FND : Outport  Tag=STV Outport  Port=12
  Snsr0FCCN : Outport  Tag=STV Outport  Port=13
  Snsr1FCCN : Outport  Tag=STV Outport  Port=14
  Snsr0ND_ID0 : Outport  Tag=STV Outport  Port=15
  Snsr1ND_ID1 : Outport  Tag=STV Outport  Port=16
  Snsr0ND : Outport  Tag=STV Outport  Port=17
  Snsr1ND : Outport  Tag=STV Outport  Port=18
  wires:
  FromWs/1 -> Demux/1
  Demux/1 -> InitTrg/1
  Demux/2 -> AutTrimSrv/1
  Demux/3 -> ClearTrimSrv/1
  Demux/4 -> ReadTrimSrv/1
  Demux/5 -> WrSrv/1
  Demux/6 -> TrimPrfmdStsSrv/1
  Demux/7 -> HwAg0OffsTrimData/1
  Demux/8 -> Polarity/1
  Demux/9 -> CSSnsr0/1
  Demux/10 -> CSSnsr1/1
  Demux/11 -> Snsr0FND/1
  Demux/12 -> Snsr1FND/1
  Demux/13 -> Snsr0FCCN/1
  Demux/14 -> Snsr1FCCN/1
  Demux/15 -> Snsr0ND_ID0/1
  Demux/16 -> Snsr1ND_ID1/1
  Demux/17 -> Snsr0ND/1
  Demux/18 -> Snsr1ND/1

== system CM690A_HwAg0Meas/HwAg0Meas/HwAg0MeasHwAg0AutTrim/CopyRight2 ==

== system CM690A_HwAg0Meas/HwAg0Meas/HwAg0MeasHwAg0ClrTrim/CopyRight2 ==

== system CM690A_HwAg0Meas/HwAg0Meas/HwAg0MeasHwAg0ReadTrim/CopyRight2 ==

== system CM690A_HwAg0Meas/HwAg0Meas/HwAg0MeasHwAg0TrimPrfmdSts/CopyRight2 ==

== system CM690A_HwAg0Meas/HwAg0Meas/HwAg0MeasHwAg0WrTrim/CopyRight2 ==

== system CM690A_HwAg0Meas/HwAg0Meas/HwAg0MeasInit1/CopyRight2 ==

== system CM690A_HwAg0Meas/HwAg0Meas/HwAg0MeasInit1/GetRefTmr1MicroSec32bit ==
  CopyRight2 : Subsystem  Description=|  mask(Copyright Information){none=on}
      | Copyright info block.                                               
      |                                                                     
      | Place copyright information at the top of every subsystem in design.
      mask prompts: none "No parameters"
      mask help: Place copyright information at the top of every subsystem in design.
      mask Display:
      | NxtrConf = 'Nexteer Confidential';
      | 
      | sys = bdroot; %handle for the current model ("system")
      | first = get_param(sys,'Created');
      | first = first(end-3:end);  %year is last four digits
      | 
      | last = get_param(sys,'LastModifiedDate');
      | if isempty(last)
      |     last = datestr(now,'yyyy');
      | else
      |     last = last(end-3:end);
      | end
      | 
      | if strcmp(first,last)
      |     fprintf('%s -- Copyright %s Nexteer',NxtrConf,first)
      | else
      |     fprintf('%s -- %s%s- %s Nexteer',NxtrConf,char(169),first,last)
      | end
  Ground : Ground
  RefTmr : Outport
  wires:
  Ground/1 -> RefTmr/1

== system CM690A_HwAg0Meas/HwAg0Meas/HwAg0MeasInit1/GetTiSpan1MicroSec32bit ==
  RefTmr : Inport
  CopyRight2 : Subsystem  Description=|  mask(Copyright Information){none=on}
      | Copyright info block.                                               
      |                                                                     
      | Place copyright information at the top of every subsystem in design.
      mask prompts: none "No parameters"
      mask help: Place copyright information at the top of every subsystem in design.
      mask Display:
      | NxtrConf = 'Nexteer Confidential';
      | 
      | sys = bdroot; %handle for the current model ("system")
      | first = get_param(sys,'Created');
      | first = first(end-3:end);  %year is last four digits
      | 
      | last = get_param(sys,'LastModifiedDate');
      | if isempty(last)
      |     last = datestr(now,'yyyy');
      | else
      |     last = last(end-3:end);
      | end
      | 
      | if strcmp(first,last)
      |     fprintf('%s -- Copyright %s Nexteer',NxtrConf,first)
      | else
      |     fprintf('%s -- %s%s- %s Nexteer',NxtrConf,char(169),first,last)
      | end
  Ground : Ground
  Terminator : Terminator
  TiSpan : Outport
  wires:
  RefTmr/1 -> Terminator/1
  Ground/1 -> TiSpan/1

== system CM690A_HwAg0Meas/HwAg0Meas/HwAg0MeasInit1/IoHwAb_SetFctPrphlHwAg0 ==
  CopyRight2 : Subsystem  Description=|  mask(Copyright Information){none=on}
      | Copyright info block.                                               
      |                                                                     
      | Place copyright information at the top of every subsystem in design.
      mask prompts: none "No parameters"
      mask help: Place copyright information at the top of every subsystem in design.
      mask Display:
      | NxtrConf = 'Nexteer Confidential';
      | 
      | sys = bdroot; %handle for the current model ("system")
      | first = get_param(sys,'Created');
      | first = first(end-3:end);  %year is last four digits
      | 
      | last = get_param(sys,'LastModifiedDate');
      | if isempty(last)
      |     last = datestr(now,'yyyy');
      | else
      |     last = last(end-3:end);
      | end
      | 
      | if strcmp(first,last)
      |     fprintf('%s -- Copyright %s Nexteer',NxtrConf,first)
      | else
      |     fprintf('%s -- %s%s- %s Nexteer',NxtrConf,char(169),first,last)
      | end

== system CM690A_HwAg0Meas/HwAg0Meas/HwAg0MeasPer1/CopyRight2 ==

== system CM690A_HwAg0Meas/HwAg0Meas/HwAg0MeasPer1/GetRefTmr1MicroSec32bit1 ==
  CopyRight2 : Subsystem  Description=|  mask(Copyright Information){none=on}
      | Copyright info block.                                               
      |                                                                     
      | Place copyright information at the top of every subsystem in design.
      mask prompts: none "No parameters"
      mask help: Place copyright information at the top of every subsystem in design.
      mask Display:
      | NxtrConf = 'Nexteer Confidential';
      | 
      | sys = bdroot; %handle for the current model ("system")
      | first = get_param(sys,'Created');
      | first = first(end-3:end);  %year is last four digits
      | 
      | last = get_param(sys,'LastModifiedDate');
      | if isempty(last)
      |     last = datestr(now,'yyyy');
      | else
      |     last = last(end-3:end);
      | end
      | 
      | if strcmp(first,last)
      |     fprintf('%s -- Copyright %s Nexteer',NxtrConf,first)
      | else
      |     fprintf('%s -- %s%s- %s Nexteer',NxtrConf,char(169),first,last)
      | end
  Ground : Ground
  RefTmr : Outport
  wires:
  Ground/1 -> RefTmr/1

== system CM690A_HwAg0Meas/HwAg0Meas/HwAg0MeasPer1/GetTiSpan1MicroSec32bit ==
  RefTmr : Inport
  CopyRight2 : Subsystem  Description=|  mask(Copyright Information){none=on}
      | Copyright info block.                                               
      |                                                                     
      | Place copyright information at the top of every subsystem in design.
      mask prompts: none "No parameters"
      mask help: Place copyright information at the top of every subsystem in design.
      mask Display:
      | NxtrConf = 'Nexteer Confidential';
      | 
      | sys = bdroot; %handle for the current model ("system")
      | first = get_param(sys,'Created');
      | first = first(end-3:end);  %year is last four digits
      | 
      | last = get_param(sys,'LastModifiedDate');
      | if isempty(last)
      |     last = datestr(now,'yyyy');
      | else
      |     last = last(end-3:end);
      | end
      | 
      | if strcmp(first,last)
      |     fprintf('%s -- Copyright %s Nexteer',NxtrConf,first)
      | else
      |     fprintf('%s -- %s%s- %s Nexteer',NxtrConf,char(169),first,last)
      | end
  Ground : Ground
  Terminator : Terminator
  TiSpan : Outport
  wires:
  RefTmr/1 -> Terminator/1
  Ground/1 -> TiSpan/1

== system CM690A_HwAg0Meas/HwAg0Meas/HwAg0MeasPer1/IncrementCount ==
  Action Port : ActionPort  ActionType=then
  Add : Sum
  Constant : Constant  OutDataTypeStr=uint8
  CopyRight2 : Subsystem  Description=|  mask(Copyright Information){none=on}
      | Copyright info block.                                               
      |                                                                     
      | Place copyright information at the top of every subsystem in design.
      mask prompts: none "No parameters"
      mask help: Place copyright information at the top of every subsystem in design.
      mask Display:
      | NxtrConf = 'Nexteer Confidential';
      | 
      | sys = bdroot; %handle for the current model ("system")
      | first = get_param(sys,'Created');
      | first = first(end-3:end);  %year is last four digits
      | 
      | last = get_param(sys,'LastModifiedDate');
      | if isempty(last)
      |     last = datestr(now,'yyyy');
      | else
      |     last = last(end-3:end);
      | end
      | 
      | if strcmp(first,last)
      |     fprintf('%s -- Copyright %s Nexteer',NxtrConf,first)
      | else
      |     fprintf('%s -- %s%s- %s Nexteer',NxtrConf,char(169),first,last)
      | end
  Data Store Read : DataStoreRead  DataStoreName=HwAg0SnsrTrigNr
  Data Store Write : DataStoreWrite  DataStoreName=HwAg0SnsrTrigNr
  wires:
  Add/1 -> Data Store Write/1
  Data Store Read/1 -> Add/1
  Constant/1 -> Add/2

== stateflow chart CM690A_HwAg0Meas/HwAg0Meas/HwAg0MeasPer2/Snsr0Read/SetNtcSts/ISO Fault Debounce Design ==
  settings: stateMachineType=MEALY_MACHINE
  note: NTCSTS_PASSD           (0)
      | NTCSTS_FAILD             (1)
      | NTCSTS_PREPASSD   (2)
      | NTCSTS_PREFAILD     (3)
      |
      | SIGQLFR_NORES        (0)
      | SIGQLFR_PASSD         (1)
      | SIGQLFR_FAILD           (2)
  note: Pass Loop
  note: Fail Loop
  note: 
  (default) -> (junction 89)
  (junction 89) -> (junction 95) [order 1] : [NtcSts ==3]
  (junction 89) -> (junction 93) [order 2] : [NtcSts ==2]
  (junction 89) -> (junction 141) [order 3] : [NtcSts ==1]
      | { ErrAcc = 32767;
      | Qualifier =2;
      |  }
  (junction 89) -> (junction 141) [order 4] : [NtcSts ==0]
      | { ErrAcc = -32768;
      | Qualifier=1;
      | }
  (junction 95) -> (junction 103) [order 2]
  (junction 95) -> (junction 111) [order 1] : [ErrAcc <=0]
      | {ErrAcc = DebStep;}
  (junction 93) -> (junction 123) [order 2] : {
      | ErrAcc = ErrAcc - DebStep;
      | }
  (junction 93) -> (junction 123) [order 1] : [(ErrAcc - DebStep) <= -32768]
      | { ErrAcc = -32768;
      | Qualifier=1;
      | }
  (junction 103) -> (junction 111) [order 1] : [(ErrAcc + DebStep) <32767]
      | {ErrAcc = ErrAcc + DebStep;}
  (junction 103) -> (junction 111) [order 2] : {ErrAcc = 32767;
      | Qualifier =2;}
  (junction 123) -> (junction 141)
  (junction 111) -> (junction 141)
  (junction 141) -> (junction 159) [order 2] : {ErrAcc = 0;
      | Qualifier =0;
      | }
  (junction 141) -> (junction 159) [order 1] : [SvcClr ==0]
  data: NtcSts input uint8; Qualifier output uint8; DebStep input uint16; ErrAcc local single; SvcClr input

== stateflow chart CM690A_HwAg0Meas/HwAg0Meas/HwAg0MeasPer3/Snsr1Read/SetNtcSts/ISO Fault Debounce Design ==
  settings: stateMachineType=MEALY_MACHINE
  note: NTCSTS_PASSD           (0)
      | NTCSTS_FAILD             (1)
      | NTCSTS_PREPASSD   (2)
      | NTCSTS_PREFAILD     (3)
      |
      | SIGQLFR_NORES        (0)
      | SIGQLFR_PASSD         (1)
      | SIGQLFR_FAILD           (2)
  note: Pass Loop
  note: Fail Loop
  note: 
  (default) -> (junction 89)
  (junction 89) -> (junction 95) [order 1] : [NtcSts ==3]
  (junction 89) -> (junction 93) [order 2] : [NtcSts ==2]
  (junction 89) -> (junction 141) [order 3] : [NtcSts ==1]
      | { ErrAcc = 32767;
      | Qualifier =2;
      |  }
  (junction 89) -> (junction 141) [order 4] : [NtcSts ==0]
      | { ErrAcc = -32768;
      | Qualifier=1;
      | }
  (junction 95) -> (junction 103) [order 2]
  (junction 95) -> (junction 111) [order 1] : [ErrAcc <=0]
      | {ErrAcc = DebStep;}
  (junction 93) -> (junction 123) [order 2] : {
      | ErrAcc = ErrAcc - DebStep;
      | }
  (junction 93) -> (junction 123) [order 1] : [(ErrAcc - DebStep) <= -32768]
      | { ErrAcc = -32768;
      | Qualifier=1;
      | }
  (junction 103) -> (junction 111) [order 1] : [(ErrAcc + DebStep) <32767]
      | {ErrAcc = ErrAcc + DebStep;}
  (junction 103) -> (junction 111) [order 2] : {ErrAcc = 32767;
      | Qualifier =2;}
  (junction 123) -> (junction 141)
  (junction 111) -> (junction 141)
  (junction 141) -> (junction 159) [order 2] : {ErrAcc = 0;
      | Qualifier =0;
      | }
  (junction 141) -> (junction 159) [order 1] : [SvcClr ==0]
  data: NtcSts input uint8; Qualifier output uint8; DebStep input uint16; ErrAcc local single; SvcClr input

== system CM690A_HwAg0Meas/HwAg0Meas/HwAg0MeasPer1/ResetCount ==
  Action Port : ActionPort  ActionType=else
  Constant1 : Constant  Value=HWAG10THTOOTHTRIG_CNT_U08
      settings: AttributesFormatString=%<Value>.EngVal = 1
  CopyRight2 : Subsystem  Description=|  mask(Copyright Information){none=on}
      | Copyright info block.                                               
      |                                                                     
      | Place copyright information at the top of every subsystem in design.
      mask prompts: none "No parameters"
      mask help: Place copyright information at the top of every subsystem in design.
      mask Display:
      | NxtrConf = 'Nexteer Confidential';
      | 
      | sys = bdroot; %handle for the current model ("system")
      | first = get_param(sys,'Created');
      | first = first(end-3:end);  %year is last four digits
      | 
      | last = get_param(sys,'LastModifiedDate');
      | if isempty(last)
      |     last = datestr(now,'yyyy');
      | else
      |     last = last(end-3:end);
      | end
      | 
      | if strcmp(first,last)
      |     fprintf('%s -- Copyright %s Nexteer',NxtrConf,first)
      | else
      |     fprintf('%s -- %s%s- %s Nexteer',NxtrConf,char(169),first,last)
      | end
  Data Store Write : DataStoreWrite  DataStoreName=HwAg0SnsrTrigNr
  wires:
  Constant1/1 -> Data Store Write/1

== system CM690A_HwAg0Meas/HwAg0Meas/HwAg0MeasPer2/CopyRight2 ==

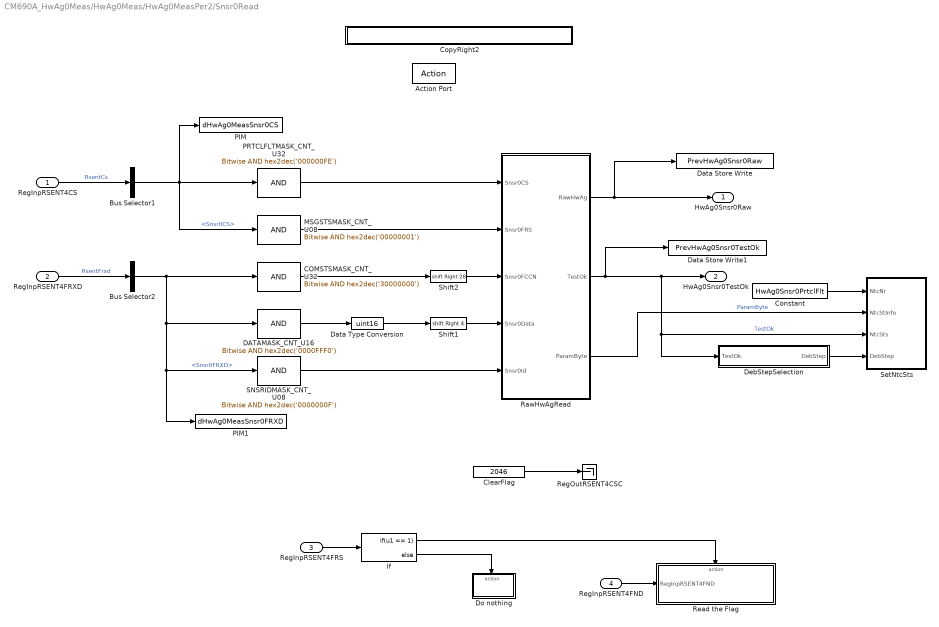
== system CM690A_HwAg0Meas/HwAg0Meas/HwAg0MeasPer2/Snsr0Read ==
  RegInpRSENT4CS : Inport
  RegInpRSENT4FRXD : Inport  Port=2
  RegInpRSENT4FRS : Inport  Port=3
  RegInpRSENT4FND : Inport  Port=4
  Action Port : ActionPort  ActionType=then
  Bus Selector1 : BusSelector  OutputSignals=Snsr0CS
  Bus Selector2 : BusSelector  OutputSignals=Snsr0FRXD
  COMSTSMASK_CNT_U32 : simulink/Logic and Bit Operations/Bitwise Operator  logicop=AND  UseBitMask=on  BitMask=hex2dec('30000000')  BitMaskRealWorld=Stored Integer
  ClearFlag : Constant  RequirementInfo={} %GIDa_57b4b637_df2c_4ddd_aec4_0c4d3893fab0  Value=2046  OutDataTypeStr=uint16
  Constant : Constant  Value=HwAg0Snsr0PrtclFlt
  CopyRight2 : Subsystem  Description=|  mask(Copyright Information){none=on}
      | Copyright info block.                                               
      |                                                                     
      | Place copyright information at the top of every subsystem in design.
      mask prompts: none "No parameters"
      mask help: Place copyright information at the top of every subsystem in design.
      mask Display:
      | NxtrConf = 'Nexteer Confidential';
      | 
      | sys = bdroot; %handle for the current model ("system")
      | first = get_param(sys,'Created');
      | first = first(end-3:end);  %year is last four digits
      | 
      | last = get_param(sys,'LastModifiedDate');
      | if isempty(last)
      |     last = datestr(now,'yyyy');
      | else
      |     last = last(end-3:end);
      | end
      | 
      | if strcmp(first,last)
      |     fprintf('%s -- Copyright %s Nexteer',NxtrConf,first)
      | else
      |     fprintf('%s -- %s%s- %s Nexteer',NxtrConf,char(169),first,last)
      | end
  DATAMASK_CNT_U16 : simulink/Logic and Bit Operations/Bitwise Operator  logicop=AND  UseBitMask=on  BitMask=hex2dec('0000FFF0')  BitMaskRealWorld=Stored Integer
  Data Store Write : DataStoreWrite  DataStoreName=PrevHwAg0Snsr0Raw
  Data Store Write1 : DataStoreWrite  DataStoreName=PrevHwAg0Snsr0TestOk
  Data Type Conversion : DataTypeConversion  OutDataTypeStr=uint16
  DebStepSelection : Subsystem
  Do nothing : Subsystem  RequirementInfo={} %GIDa_9056e706_3d71_4a53_915e_13e7349e7ef8  TreatAsAtomicUnit=on
  If : If  RequirementInfo={} %GIDa_f8157777_8e5c_4d0f_87bb_de1a0d69ea62  IfExpression=u1 == 1
  MSGSTSMASK_CNT_U08 : simulink/Logic and Bit Operations/Bitwise Operator  logicop=AND  UseBitMask=on  BitMask=hex2dec('00000001')  BitMaskRealWorld=Stored Integer
  PIM : DataStoreWrite  RequirementInfo={} %GIDa_1caef41a_c931_4b50_b2a9_baea7ac55603  DataStoreName=dHwAg0MeasSnsr0CS
  PIM1 : DataStoreWrite  RequirementInfo={} %GIDa_993a9dff_4859_40a5_8744_cc08ea3de3d6  DataStoreName=dHwAg0MeasSnsr0FRXD
  PRTCLFLTMASK_CNT_U32 : simulink/Logic and Bit Operations/Bitwise Operator  logicop=AND  UseBitMask=on  BitMask=hex2dec('000000FE')  BitMaskRealWorld=Stored Integer
  RawHwAgRead : Subsystem  RequirementInfo={'linktype_rmi_doors' '0000cf45 (/ESG Group/FDD Module Requirements/EA4 Specific/CM690A_HwAg0Meas)' '#CM690A_27' 'true' 'REQ: CM690A_27' '' } %GIDa_f7aa6691_9a65_4843_8cfe_9a20ed5db07a
  Read the Flag : Subsystem  RequirementInfo={} %GIDa_f340db1e_b823_47e1_bbd3_bfc14f49b8cf  TreatAsAtomicUnit=on
  RegOutRSENT4CSC : Terminator
  SNSRIDMASK_CNT_U08 : simulink/Logic and Bit Operations/Bitwise Operator  logicop=AND  UseBitMask=on  BitMask=hex2dec('0000000F')  BitMaskRealWorld=Stored Integer
  SetNtcSts : Subsystem  RequirementInfo={'linktype_rmi_doors' '0000cf45 (/ESG Group/FDD Module Requirements/EA4 Specific/CM690A_HwAg0Meas)' '#CM690A_38' 'true' 'REQ: CM690A_38' '' } %GIDa_5188fc61_ece4_46a3_bf12_39d3cc555501
  Shift1 : ArithShift  BitShiftNumber=4  BitShiftDirection=Right
  Shift2 : ArithShift  BitShiftNumber=28  BitShiftDirection=Right
  HwAg0Snsr0Raw : Outport
  HwAg0Snsr0TestOk : Outport  Port=2
  wires:
  RawHwAgRead/2(TestOk) -> Data Store Write1/1, DebStepSelection/1(TestOk), SetNtcSts/3(NtcSts), HwAg0Snsr0TestOk/1  "TestOk"
  RawHwAgRead/3(ParamByte) -> SetNtcSts/2(NtcStInfo)  "ParamByte"
  DebStepSelection/1(DebStep) -> SetNtcSts/4(DebStep)
  Constant/1 -> SetNtcSts/1(NtcNr)
  RawHwAgRead/1(RawHwAg) -> Data Store Write/1, HwAg0Snsr0Raw/1
  RegInpRSENT4CS/1 -> Bus Selector1/1  "RsentCs"
  PRTCLFLTMASK_CNT_U32/1 -> RawHwAgRead/1(Snsr0CS)
  MSGSTSMASK_CNT_U08/1 -> RawHwAgRead/2(Snsr0FRS)
  COMSTSMASK_CNT_U32/1 -> Shift2/1
  RegInpRSENT4FRXD/1 -> Bus Selector2/1  "RsentFrxd"
  DATAMASK_CNT_U16/1 -> Data Type Conversion/1
  SNSRIDMASK_CNT_U08/1 -> RawHwAgRead/5(Snsr0Id)
  Shift1/1 -> RawHwAgRead/4(Snsr0Data)
  Shift2/1 -> RawHwAgRead/3(Snsr0FCCN)
  Bus Selector1/1 -> PIM/1, MSGSTSMASK_CNT_U08/1, PRTCLFLTMASK_CNT_U32/1  "<Snsr0CS>"
  Bus Selector2/1 -> PIM1/1, SNSRIDMASK_CNT_U08/1, DATAMASK_CNT_U16/1, COMSTSMASK_CNT_U32/1  "<Snsr0FRXD>"
  Data Type Conversion/1 -> Shift1/1
  ClearFlag/1 -> RegOutRSENT4CSC/1
  RegInpRSENT4FRS/1 -> If/1
  If/1 -> Read the Flag/Action
  If/2 -> Do nothing/Action
  RegInpRSENT4FND/1 -> Read the Flag/1(RegInpRSENT4FND)

== system CM690A_HwAg0Meas/HwAg0Meas/HwAg0MeasPer2/Snsr0Read1 ==
  Action Port : ActionPort  ActionType=else
  CopyRight2 : Subsystem  Description=|  mask(Copyright Information){none=on}
      | Copyright info block.                                               
      |                                                                     
      | Place copyright information at the top of every subsystem in design.
      mask prompts: none "No parameters"
      mask help: Place copyright information at the top of every subsystem in design.
      mask Display:
      | NxtrConf = 'Nexteer Confidential';
      | 
      | sys = bdroot; %handle for the current model ("system")
      | first = get_param(sys,'Created');
      | first = first(end-3:end);  %year is last four digits
      | 
      | last = get_param(sys,'LastModifiedDate');
      | if isempty(last)
      |     last = datestr(now,'yyyy');
      | else
      |     last = last(end-3:end);
      | end
      | 
      | if strcmp(first,last)
      |     fprintf('%s -- Copyright %s Nexteer',NxtrConf,first)
      | else
      |     fprintf('%s -- %s%s- %s Nexteer',NxtrConf,char(169),first,last)
      | end
  Data Store Read : DataStoreRead  DataStoreName=PrevHwAg0Snsr0Raw
  Data Store Read1 : DataStoreRead  DataStoreName=PrevHwAg0Snsr0TestOk
  HwAg0Snsr0Raw : Outport
  HwAg0Snsr0TestOk : Outport  Port=2
  wires:
  Data Store Read/1 -> HwAg0Snsr0Raw/1
  Data Store Read1/1 -> HwAg0Snsr0TestOk/1

== system CM690A_HwAg0Meas/HwAg0Meas/HwAg0MeasPer3/CopyRight2 ==

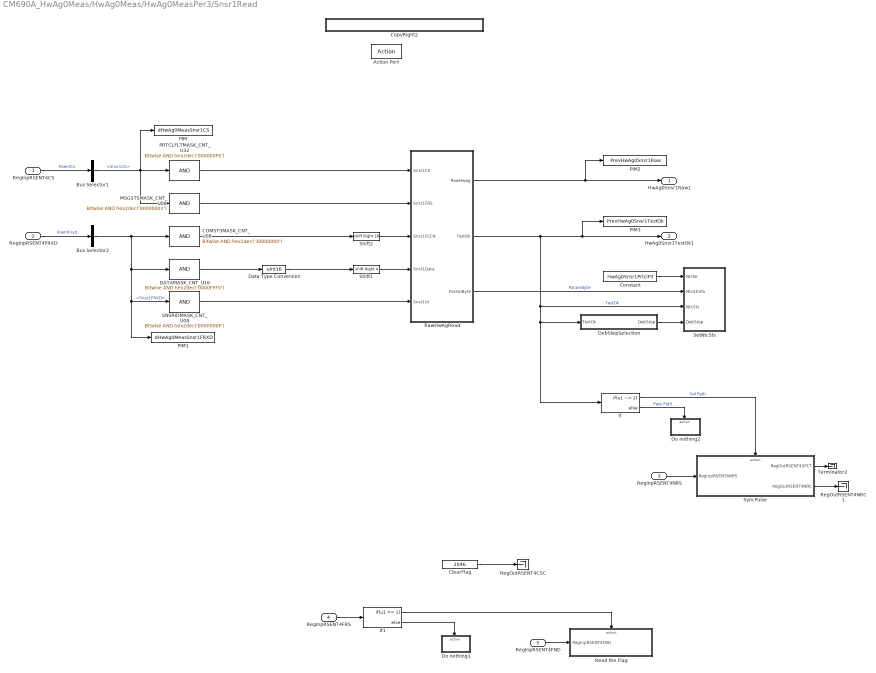
== system CM690A_HwAg0Meas/HwAg0Meas/HwAg0MeasPer3/Snsr1Read ==
  RegInpRSENT4CS : Inport
  RegInpRSENT4FRXD : Inport  Port=2
  RegInpRSENT4NRS : Inport  Port=3
  RegInpRSENT4FRS : Inport  Port=4
  RegInpRSENT4FND : Inport  Port=5
  Action Port : ActionPort  ActionType=then
  Bus Selector1 : BusSelector  OutputSignals=Snsr1CS
  Bus Selector2 : BusSelector  OutputSignals=Snsr1FRXD
  COMSTSMASK_CNT_U08 : simulink/Logic and Bit Operations/Bitwise Operator  logicop=AND  UseBitMask=on  BitMask=hex2dec('30000000')  BitMaskRealWorld=Stored Integer
  ClearFlag : Constant  RequirementInfo={} %GIDa_4661b7cc_311d_43df_bbef_a8b28e3c9494  Value=2046  OutDataTypeStr=uint16
  Constant : Constant  Value=HwAg0Snsr1PrtclFlt
  CopyRight2 : Subsystem  Description=|  mask(Copyright Information){none=on}
      | Copyright info block.                                               
      |                                                                     
      | Place copyright information at the top of every subsystem in design.
      mask prompts: none "No parameters"
      mask help: Place copyright information at the top of every subsystem in design.
      mask Display:
      | NxtrConf = 'Nexteer Confidential';
      | 
      | sys = bdroot; %handle for the current model ("system")
      | first = get_param(sys,'Created');
      | first = first(end-3:end);  %year is last four digits
      | 
      | last = get_param(sys,'LastModifiedDate');
      | if isempty(last)
      |     last = datestr(now,'yyyy');
      | else
      |     last = last(end-3:end);
      | end
      | 
      | if strcmp(first,last)
      |     fprintf('%s -- Copyright %s Nexteer',NxtrConf,first)
      | else
      |     fprintf('%s -- %s%s- %s Nexteer',NxtrConf,char(169),first,last)
      | end
  DATAMASK_CNT_U16 : simulink/Logic and Bit Operations/Bitwise Operator  logicop=AND  UseBitMask=on  BitMask=hex2dec('0000FFF0')  BitMaskRealWorld=Stored Integer
  Data Type Conversion : DataTypeConversion  OutDataTypeStr=uint16
  DebStepSelection : Subsystem
  Do nothing1 : Subsystem  RequirementInfo={} %GIDa_85580e43_c8a5_4380_a97a_a9810241ddad  TreatAsAtomicUnit=on
  Do nothing2 : Subsystem  RequirementInfo={} %GIDa_b8c0d833_a855_4970_b781_b9a37ee5f01a  TreatAsAtomicUnit=on
  If : If  RequirementInfo={} %GIDa_9d788ab9_4eec_425d_ae52_01f7ab9715c5  IfExpression=u1 ~= 2
  If1 : If  RequirementInfo={} %GIDa_1ded9a8e_35f8_478c_9d47_9bfc346c5efa  IfExpression=u1 == 1
  MSGSTSMASK_CNT_U08 : simulink/Logic and Bit Operations/Bitwise Operator  logicop=AND  UseBitMask=on  BitMask=hex2dec('00000001')  BitMaskRealWorld=Stored Integer
  PIM : DataStoreWrite  RequirementInfo={} %GIDa_75ad949c_ec95_4341_a392_745e55ce9a03  DataStoreName=dHwAg0MeasSnsr1CS
  PIM1 : DataStoreWrite  RequirementInfo={} %GIDa_d85a10da_f47e_48f8_9150_fb3481b8223f  DataStoreName=dHwAg0MeasSnsr1FRXD
  PIM2 : DataStoreWrite  RequirementInfo={} %GIDa_1878a1c5_af77_4885_ae52_51d7bb7c8c9f  DataStoreName=PrevHwAg0Snsr1Raw
  PIM3 : DataStoreWrite  RequirementInfo={} %GIDa_a019fdda_c21f_4ce1_ba75_99decb5deb9d  DataStoreName=PrevHwAg0Snsr1TestOk
  PRTCLFLTMASK_CNT_U32 : simulink/Logic and Bit Operations/Bitwise Operator  logicop=AND  UseBitMask=on  BitMask=hex2dec('000000FE')  BitMaskRealWorld=Stored Integer
  RawHwAgRead : Subsystem  RequirementInfo={'linktype_rmi_doors' '0000cf45 (/ESG Group/FDD Module Requirements/EA4 Specific/CM690A_HwAg0Meas)' '#CM690A_27' 'true' 'REQ: CM690A_27' '' } %GIDa_159a886d_48a1_43f3_ac64_8292abeb2afb
  Read the Flag : Subsystem  RequirementInfo={} %GIDa_bf8cb5e8_96d2_4b62_8d28_543f7f7ca925  TreatAsAtomicUnit=on
  RegOutRSENT4CSC : Terminator
  RegOutRSENT4NRC1 : Terminator
  SNSRIDMASK_CNT_U08 : simulink/Logic and Bit Operations/Bitwise Operator  logicop=AND  UseBitMask=on  BitMask=hex2dec('0000000F')  BitMaskRealWorld=Stored Integer
  SetNtcSts : Subsystem  RequirementInfo={'linktype_rmi_doors' '0000cf45 (/ESG Group/FDD Module Requirements/EA4 Specific/CM690A_HwAg0Meas)' '#CM690A_53' 'true' 'REQ: CM690A_53' '' } %GIDa_6fae1fe1_05c7_41c6_87b4_f7be9d83a9d8
  Shift1 : ArithShift  BitShiftNumber=4  BitShiftDirection=Right
  Shift2 : ArithShift  BitShiftNumber=28  BitShiftDirection=Right
  SyncPulse : Subsystem  RequirementInfo={} %GIDa_a907105d_33cc_416a_acd5_75fa42c63a40  TreatAsAtomicUnit=on
  Terminator2 : Terminator
  HwAg0Snsr1Raw1 : Outport
  HwAg0Snsr1TestOk1 : Outport  Port=2
  wires:
  RawHwAgRead/2(TestOk) -> PIM3/1, HwAg0Snsr1TestOk1/1, SetNtcSts/3(NtcSts), If/1, DebStepSelection/1(TestOk)  "TestOk"
  RawHwAgRead/3(ParamByte) -> SetNtcSts/2(NtcStInfo)  "ParamByte"
  DebStepSelection/1(DebStep) -> SetNtcSts/4(DebStep)
  Constant/1 -> SetNtcSts/1(NtcNr)
  RawHwAgRead/1(RawHwAg) -> PIM2/1, HwAg0Snsr1Raw1/1
  RegInpRSENT4CS/1 -> Bus Selector1/1  "RsentCs"
  PRTCLFLTMASK_CNT_U32/1 -> RawHwAgRead/1(Snsr1CS)
  MSGSTSMASK_CNT_U08/1 -> RawHwAgRead/2(Snsr1FRS)
  COMSTSMASK_CNT_U08/1 -> Shift2/1
  RegInpRSENT4FRXD/1 -> Bus Selector2/1  "RsentFrxd"
  DATAMASK_CNT_U16/1 -> Data Type Conversion/1
  SNSRIDMASK_CNT_U08/1 -> RawHwAgRead/5(Snsr1Id)
  Shift1/1 -> RawHwAgRead/4(Snsr1Data)
  Shift2/1 -> RawHwAgRead/3(Snsr1FCCN)
  Bus Selector2/1 -> PIM1/1, SNSRIDMASK_CNT_U08/1, DATAMASK_CNT_U16/1, COMSTSMASK_CNT_U08/1  "<Snsr1FRXD>"
  Bus Selector1/1 -> PIM/1, MSGSTSMASK_CNT_U08/1, PRTCLFLTMASK_CNT_U32/1  "<Snsr1CS>"
  Data Type Conversion/1 -> Shift1/1
  If/1 -> SyncPulse/Action  "fail Path"
  If/2 -> Do nothing2/Action  "Pass Path"
  SyncPulse/1(RegOutRSENT4SPCT) -> Terminator2/1
  SyncPulse/2(RegOutRSENT4NRC) -> RegOutRSENT4NRC1/1
  RegInpRSENT4NRS/1 -> SyncPulse/1(RegInpRSENT4NRS)
  ClearFlag/1 -> RegOutRSENT4CSC/1
  RegInpRSENT4FRS/1 -> If1/1
  If1/1 -> Read the Flag/Action
  If1/2 -> Do nothing1/Action
  RegInpRSENT4FND/1 -> Read the Flag/1(RegInpRSENT4FND)

== system CM690A_HwAg0Meas/HwAg0Meas/HwAg0MeasPer3/Snsr1Read1 ==
  Action Port : ActionPort  ActionType=else
  CopyRight2 : Subsystem  Description=|  mask(Copyright Information){none=on}
      | Copyright info block.                                               
      |                                                                     
      | Place copyright information at the top of every subsystem in design.
      mask prompts: none "No parameters"
      mask help: Place copyright information at the top of every subsystem in design.
      mask Display:
      | NxtrConf = 'Nexteer Confidential';
      | 
      | sys = bdroot; %handle for the current model ("system")
      | first = get_param(sys,'Created');
      | first = first(end-3:end);  %year is last four digits
      | 
      | last = get_param(sys,'LastModifiedDate');
      | if isempty(last)
      |     last = datestr(now,'yyyy');
      | else
      |     last = last(end-3:end);
      | end
      | 
      | if strcmp(first,last)
      |     fprintf('%s -- Copyright %s Nexteer',NxtrConf,first)
      | else
      |     fprintf('%s -- %s%s- %s Nexteer',NxtrConf,char(169),first,last)
      | end
  Data Store Read : DataStoreRead  DataStoreName=PrevHwAg0Snsr1Raw
  Data Store Read1 : DataStoreRead  DataStoreName=PrevHwAg0Snsr1TestOk
  HwAg0Snsr1Raw : Outport
  HwAg0Snsr1TestOk : Outport  Port=2
  wires:
  Data Store Read/1 -> HwAg0Snsr1Raw/1
  Data Store Read1/1 -> HwAg0Snsr1TestOk/1

== system CM690A_HwAg0Meas/HwAg0Meas/HwAg0MeasPer4/CopyRight2 ==

== system CM690A_HwAg0Meas/HwAg0Meas/HwAg0MeasPer4/HwAgPrevRead ==
  Action Port : ActionPort  ActionType=else
  CopyRight2 : Subsystem  Description=|  mask(Copyright Information){none=on}
      | Copyright info block.                                               
      |                                                                     
      | Place copyright information at the top of every subsystem in design.
      mask prompts: none "No parameters"
      mask help: Place copyright information at the top of every subsystem in design.
      mask Display:
      | NxtrConf = 'Nexteer Confidential';
      | 
      | sys = bdroot; %handle for the current model ("system")
      | first = get_param(sys,'Created');
      | first = first(end-3:end);  %year is last four digits
      | 
      | last = get_param(sys,'LastModifiedDate');
      | if isempty(last)
      |     last = datestr(now,'yyyy');
      | else
      |     last = last(end-3:end);
      | end
      | 
      | if strcmp(first,last)
      |     fprintf('%s -- Copyright %s Nexteer',NxtrConf,first)
      | else
      |     fprintf('%s -- %s%s- %s Nexteer',NxtrConf,char(169),first,last)
      | end
  Data Store Read : DataStoreRead  DataStoreName=PrevHwAg0
  Data Store Read1 : DataStoreRead  DataStoreName=HwAg0PrevRollCnt
  Data Store Read2 : DataStoreRead  DataStoreName=PrevHwAg0Qlfr
  HwAg0 : Outport  RequirementInfo={} %GIDa_2a04fa0d_8906_4864_b317_b58a2bd680e6
  HwAg0Qlfr : Outport  RequirementInfo={'linktype_rmi_doors' '0000cf45 (/ESG Group/FDD Module Requirements/EA4 Specific/CM690A_HwAg0Meas)' '#CM690A_30' 'true' 'REQ: CM690A_30' '' } %GIDa_484d5b89_f3e2_43cb_ab63_4c28e6abd7dd  Port=2
  HwAg0RollgCntr : Outport  RequirementInfo={'linktype_rmi_doors' '0000cf45 (/ESG Group/FDD Module Requirements/EA4 Specific/CM690A_HwAg0Meas)' '#CM690A_31' 'true' 'REQ: CM690A_31' '' } %GIDa_255a438a_78f4_413b_ba6a_8efbb79cdd47  Port=3
  wires:
  Data Store Read/1 -> HwAg0/1
  Data Store Read1/1 -> HwAg0RollgCntr/1
  Data Store Read2/1 -> HwAg0Qlfr/1
